simulink model "DTC_Switching"  (R2014a)
settings: Solver=VariableStepDiscrete  StartTime=0.0  StopTime=1  RelTol=1e-3
libraries: powerlib x9, powerlib_meascontrol x1
settings Model: Creator=ninad gaikawad  LastModifiedBy=ninad gaikawad
settings SolverCC: ZeroCrossAlgorithm=Adaptive

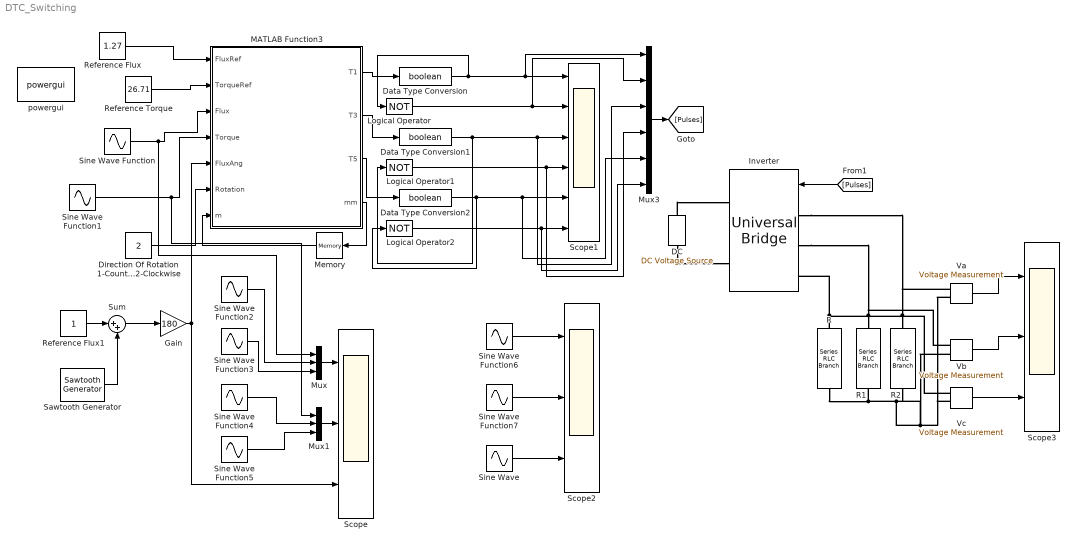
== system DTC_Switching ==
  "DC " : powerlib/Electrical Sources/DC Voltage Source  Amplitude=200  Measurements=None
  Data Type Conversion : DataTypeConversion  OutDataTypeStr=boolean
  Data Type Conversion1 : DataTypeConversion  OutDataTypeStr=boolean
  Data Type Conversion2 : DataTypeConversion  OutDataTypeStr=boolean
  Direction Of Rotation 1-CounterClockwise 2-Clockwise : Constant  Value=2
  Gain : Gain  Gain=180
  Inverter : powerlib/Power Electronics/Universal Bridge  Arms=3  SnubberResistance=1e5  SnubberCapacitance=inf  Device=IGBT / Diodes  Ron=1e-3  Lon=0  ForwardVoltages="[  0  0  ]"  ForwardVoltage=0  GTOparameters=[ 10e-6 , 20e-6 ]  IGBTparameters=[ 1e-6 , 2e-6 ]  Measurements=None  Measurements_2=None  converterType=Rectifier
  Logical Operator : Logic  Operator=NOT  AllPortsSameDT=off  OutDataTypeStr=boolean
  Logical Operator1 : Logic  Operator=NOT  AllPortsSameDT=off  OutDataTypeStr=boolean
  Logical Operator2 : Logic  Operator=NOT  AllPortsSameDT=off  OutDataTypeStr=boolean
  MATLAB Function3 : MATLAB Function  TreatAsAtomicUnit=on
  Memory : Memory  X0=1
  Mux : Mux  Inputs=3
  Mux1 : Mux  Inputs=3
  Mux3 : Mux  Inputs=6
  R : powerlib/Elements/Series RLC Branch  LConnTagsString=__new0  RConnTagsString=__new0  BranchType=R  Resistance=1000  Inductance=1e-3  SetiL0=off  InitialCurrent=0  Capacitance=1e-6  Setx0=off  InitialVoltage=0  Measurements=None
  R1 : powerlib/Elements/Series RLC Branch  LConnTagsString=__new0  RConnTagsString=__new0  BranchType=R  Resistance=1000  Inductance=1e-3  SetiL0=off  InitialCurrent=0  Capacitance=1e-6  Setx0=off  InitialVoltage=0  Measurements=None
  R2 : powerlib/Elements/Series RLC Branch  LConnTagsString=__new0  RConnTagsString=__new0  BranchType=R  Resistance=1000  Inductance=1e-3  SetiL0=off  InitialCurrent=0  Capacitance=1e-6  Setx0=off  InitialVoltage=0  Measurements=None
  Reference Flux : Constant  Value=1.27
  Reference Flux1 : Constant
  Reference Torque : Constant  Value=26.71
  Sawtooth Generator : powerlib_meascontrol/Pulse & Signal Generators/Sawtooth Generator  Freq=50  Phase=0  Ts=0
  Scope : Scope  NumInputPorts=3
      settings: YMin=-5~-5~-5  YMax=5~5~5
  Scope1 : Scope  NumInputPorts=6
      settings: YMin=-5~-5~-5~-5~-5~-5  YMax=5~5~5~5~5~5
  Scope2 : Scope  NumInputPorts=3
      settings: YMin=-5~-5~-5  YMax=5~5~5  SaveName=ScopeData2
  Scope3 : Scope  NumInputPorts=3
      settings: YMin=-5~-5~-5  YMax=5~5~5  SaveName=ScopeData3
  Sine Wave : Sin  Frequency=2*pi*50  SampleTime=0
  Sine Wave Function : Sin  Amplitude=1.3  Bias=1.27  Frequency=2*pi*50  SampleTime=0
  Sine Wave Function1 : Sin  Amplitude=28  Bias=26.71  Frequency=2*pi*50  SampleTime=0
  Sine Wave Function2 : Sin  Amplitude=1.3+0.025  Bias=1.27+0.025  Frequency=2*pi*50  SampleTime=0
  Sine Wave Function3 : Sin  Amplitude=1.3-0.025  Bias=1.27-0.025  Frequency=2*pi*50  SampleTime=0
  Sine Wave Function4 : Sin  Amplitude=26.71+0.25  Bias=26.71+0.25  Frequency=2*pi*50  SampleTime=0
  Sine Wave Function5 : Sin  Amplitude=26.71-0.25  Bias=26.71-0.25  Frequency=2*pi*50  SampleTime=0
  Sine Wave Function6 : Sin  Amplitude=1.3  Bias=1.27  Frequency=2*pi*50  SampleTime=0
  Sine Wave Function7 : Sin  Amplitude=28  Bias=26.71  Frequency=2*pi*50  SampleTime=0
  Sum : Sum  Inputs=|++
  Va : powerlib/Measurements/Voltage Measurement  PhasorSimulation=off  OutputType=Complex  PSBequivalent=0
  Vb : powerlib/Measurements/Voltage Measurement  PhasorSimulation=off  OutputType=Complex  PSBequivalent=0
  Vc : powerlib/Measurements/Voltage Measurement  PhasorSimulation=off  OutputType=Complex  PSBequivalent=0
  powergui : powerlib/powergui  Priority=1  SimulationMode=Discrete  SolverType=Tustin  SampleTime=50e-6  frequency=60  SPID=off  DisableSnubberDevices=off  DisableRonSwitches=off  DisableVfSwitches=off  SwTol=0  Interpol=off  DisplayEquations=off  Ts=0  methode=off  frequencyindice=0  Pbase=100e6  ErrMax=1e-4  Iterations=50  UnitsV=kV  UnitsW=MW  FunctionMessages=off  echomessages=off  HookPort=off  EnableUseOfTLC=off  x0status=blocks  RestoreLinks=warning  ResistiveCurrentMeasurement=off  Frange=[0:2:500]  Ylog=off  Xlog=on  ShowGrid=off  save=off  variable=ZData  structure=0  ZoomFFT=off  StartTime=0.0  cycles=1  DisplayStyle=1  fundamental=60  FreqAxis=off  MaxFrequency=1000  frequencyindicesteady=1  RmsSteady=1  display=off
  wires:
  Sine Wave Function/1 -> Mux/1, MATLAB Function3/3(Flux)
  Sine Wave Function1/1 -> MATLAB Function3/4(Torque), Mux1/1
  Reference Flux/1 -> MATLAB Function3/1(FluxRef)
  Reference Torque/1 -> MATLAB Function3/2(TorqueRef)
  Direction Of Rotation 1-CounterClockwise 2-Clockwise/1 -> MATLAB Function3/6(Rotation)
  MATLAB Function3/1(T1) -> Data Type Conversion/1
  MATLAB Function3/2(T3) -> Data Type Conversion1/1
  MATLAB Function3/3(T5) -> Data Type Conversion2/1
  Logical Operator/1 -> Mux3/2, Scope1/2
  Logical Operator2/1 -> Mux3/6, Scope1/6
  Data Type Conversion/1 -> Logical Operator/1, Mux3/1, Scope1/1
  Data Type Conversion2/1 -> Logical Operator2/1, Mux3/5, Scope1/5
  Data Type Conversion1/1 -> Logical Operator1/1, Mux3/3, Scope1/3
  MATLAB Function3/4(mm) -> Memory/1
  Memory/1 -> MATLAB Function3/7(m)
  Reference Flux1/1 -> Sum/1
  Sawtooth Generator/1 -> Sum/2
  Sum/1 -> Gain/1
  Gain/1 -> MATLAB Function3/5(FluxAng), Scope/3
  Mux/1 -> Scope/1
  Mux1/1 -> Scope/2
  Sine Wave Function2/1 -> Mux/2
  Sine Wave Function3/1 -> Mux/3
  Sine Wave Function4/1 -> Mux1/2
  Sine Wave Function5/1 -> Mux1/3
  Sine Wave Function7/1 -> Scope2/2
  Sine Wave Function6/1 -> Scope2/1
  Sine Wave/1 -> Scope2/3
  Va/1 -> Scope3/1
  Vb/1 -> Scope3/2
  Vc/1 -> Scope3/3
  Logical Operator1/1 -> Mux3/4, Scope1/4
  [Pulses] -> Inverter/1
  Mux3/1 -> [Pulses]
  connections:
  Vc/LConn1 -- R/LConn1 -- Inverter/LConn3
  R1/LConn1 -- Inverter/LConn2 -- Vb/LConn1
  R2/LConn1 -- Inverter/LConn1 -- Va/LConn1
  R1/RConn1 -- R/RConn1 -- R2/RConn1 -- Vb/LConn2 -- Va/LConn2 -- Vc/LConn2
  "DC "/RConn1 -- Inverter/RConn1
  "DC "/LConn1 -- Inverter/RConn2

== matlab function DTC_Switching/MATLAB Function3 ==
  settings: updateMethod=CONTINUOUS
  data: FluxRef input; TorqueRef input; Flux input; Torque input; T1 output; T3 output; FluxAng input; T5 output; Rotation input; m input; mm output
function [T1,T3,T5,mm] = DTC_SwitchingTable(FluxRef,TorqueRef,Flux,Torque,FluxAng,Rotation,m)
 
T1=0;
T3=0;
T5=0;

DelF=0.025;% Hysteresis Width for Flux
DelT=0.25;% Hysteresis Width for Torque

Hf=0;%Initializing Hysteresis Controller Output For Flux
Ht=0;%Initializing Hysteresis Controller Output For Torque
S=0;%Initializing DTC Space Vector Sector
mm=m;
% Flux Two Level Hysteresis Band %
%------------------------------------------------------------------------%
if(Flux<=(FluxRef-DelF))
    Hf=1;
    mm=Hf;
end
if(mm==1&&(Flux>(FluxRef-DelF)&&Flux<(FluxRef+DelF)))
    Hf=1;
    mm=Hf;
end
if(Flux>=(FluxRef+DelF))
    Hf=0;
    mm=Hf;
end
if(mm==0&&(Flux>(FluxRef-DelF)&&Flux<(FluxRef+DelF)))
    Hf=0;
    mm=Hf;
end

% Torque Three Level Hysteresis Band %
%------------------------------------------------------------------------%
if(Torque<=(TorqueRef-DelT))
    Ht=1;
end
if(Torque>(TorqueRef-DelT)&&Torque<(TorqueRef+DelT))
    Ht=0;
end
if(Torque>=(TorqueRef+DelT))
    Ht=-1;
end

% DTC Sector Prediction %
%------------------------------------------------------------------------%
if(FluxAng>=330&&FluxAng<30)
    S=1;
end
if(FluxAng>=30&&FluxAng<90)
    S=2;
end
if(FluxAng>=90&&FluxAng<150)
    S=3;
end
if(FluxAng>=150&&FluxAng<210)
    S=4;
end
if(FluxAng>=210&&FluxAng<270)
    S=5;
end
if(FluxAng>=270&&FluxAng<330)
    S=6;
end

% Voltage Vector Synthesis %
%------------------------------------------------------------------------%
if(Rotation==2)% Clockwise Rotation
%------------------------------------------------------------------------%    
    if(Hf==1&&Ht==1&&S==1)
        T1=1;
        T3=0;
        T5=1;
    end
    if(Hf==1&&Ht==1&&S==2)
      T1=0;
      T3=0;
      T5=1;  
    end
    if(Hf==1&&Ht==1&&S==3)
      T1=0;
      T3=1;
      T5=1; 
    end
    if(Hf==1&&Ht==1&&S==4)
      T1=0;
      T3=1;
      T5=0;
    end
    if(Hf==1&&Ht==1&&S==5)
      T1=1;
      T3=1;
      T5=0;    
    end
    if(Hf==1&&Ht==1&&S==6)
      T1=1;
      T3=0;
      T5=0;
    end
   
%------------------------------------------------------------------------%    
    if(Hf==1&&Ht==0&&S==1)
        T1=1;
        T3=1;
        T5=1;
    end
    if(Hf==1&&Ht==0&&S==2)
      T1=0;
      T3=0;
      T5=0;  
    end
    if(Hf==1&&Ht==0&&S==3)
      T1=1;
      T3=1;
      T5=1; 
    end
    if(Hf==1&&Ht==0&&S==4)
      T1=0;
      T3=0;
      T5=0;
    end
    if(Hf==1&&Ht==0&&S==5)
      T1=1;
      T3=1;
      T5=1;    
    end
    if(Hf==1&&Ht==0&&S==6)
      T1=0;
      T3=0;
      T5=0;
    end
%------------------------------------------------------------------------%    
    if(Hf==1&&Ht==-1&&S==1)
        T1=1;
        T3=1;
        T5=0;
    end
    if(Hf==1&&Ht==-1&&S==2)
      T1=1;
      T3=0;
      T5=0;  
    end
    if(Hf==1&&Ht==-1&&S==3)
      T1=1;
      T3=0;
      T5=1; 
    end
    if(Hf==1&&Ht==-1&&S==4)
      T1=0;
      T3=0;
      T5=1;
    end
    if(Hf==1&&Ht==-1&&S==5)
      T1=0;
      T3=1;
      T5=1;    
    end
    if(Hf==1&&Ht==-1&&S==6)
      T1=0;
      T3=1;
      T5=0;
    end
    
 %------------------------------------------------------------------------%   
    
     if(Hf==0&&Ht==1&&S==1)
        T1=0;
        T3=0;
        T5=1;
    end
    if(Hf==0&&Ht==1&&S==2)
      T1=0;
      T3=1;
      T5=1;  
    end
    if(Hf==0&&Ht==1&&S==3)
      T1=0;
      T3=1;
      T5=0; 
    end
    if(Hf==0&&Ht==1&&S==4)
      T1=1;
      T3=1;
      T5=0;
    end
    if(Hf==0&&Ht==1&&S==5)
      T1=1;
      T3=0;
      T5=0;    
    end
    if(Hf==0&&Ht==1&&S==6)
      T1=1;
      T3=0;
      T5=1;
    end
%------------------------------------------------------------------------%    
    
    if(Hf==0&&Ht==0&&S==1)
        T1=0;
        T3=0;
        T5=0;
    end
    if(Hf==0&&Ht==0&&S==2)
      T1=1;
      T3=1;
      T5=1;  
    end
    if(Hf==0&&Ht==0&&S==3)
      T1=0;
      T3=0;
      T5=0; 
    end
    if(Hf==0&&Ht==0&&S==4)
      T1=1;
      T3=1;
      T5=1;
    end
    if(Hf==0&&Ht==0&&S==5)
      T1=0;
      T3=0;
      T5=0;    
    end
    if(Hf==0&&Ht==0&&S==6)
      T1=1;
      T3=1;
      T5=1;
    end
  %------------------------------------------------------------------------%  
    
    if(Hf==0&&Ht==-1&&S==1)
        T1=0;
        T3=1;
        T5=0;
    end
    if(Hf==0&&Ht==-1&&S==2)
      T1=1;
      T3=1;
      T5=0;  
    end
    if(Hf==0&&Ht==-1&&S==3)
      T1=1;
      T3=0;
      T5=0; 
    end
    if(Hf==0&&Ht==-1&&S==4)
      T1=1;
      T3=0;
      T5=1;
    end
    if(Hf==0&&Ht==-1&&S==5)
      T1=0;
      T3=0;
      T5=1;    
    end
    if(Hf==0&&Ht==-1&&S==6)
      T1=0;
      T3=1;
      T5=1;
    end
end

%------------------------------------------------------------------------%
if(Rotation==1)% Counter-Clockwise Rotation
%------------------------------------------------------------------------%    
    if(Hf==1&&Ht==1&&S==1)
        T1=1;
        T3=1;
        T5=0;
    end
    if(Hf==1&&Ht==1&&S==2)
      T1=0;
      T3=1;
      T5=0;  
    end
    if(Hf==1&&Ht==1&&S==3)
      T1=0;
      T3=1;
      T5=1; 
    end
    if(Hf==1&&Ht==1&&S==4)
      T1=0;
      T3=0;
      T5=1;
    end
    if(Hf==1&&Ht==1&&S==5)
      T1=1;
      T3=0;
      T5=1;    
    end
    if(Hf==1&&Ht==1&&S==6)
      T1=1;
      T3=0;
      T5=0;
    end
   
%------------------------------------------------------------------------%    
    if(Hf==1&&Ht==0&&S==1)
        T1=1;
        T3=1;
        T5=1;
    end
    if(Hf==1&&Ht==0&&S==2)
      T1=0;
      T3=0;
      T5=0;  
    end
    if(Hf==1&&Ht==0&&S==3)
      T1=1;
      T3=1;
      T5=1; 
    end
    if(Hf==1&&Ht==0&&S==4)
      T1=0;
      T3=0;
      T5=0;
    end
    if(Hf==1&&Ht==0&&S==5)
      T1=1;
      T3=1;
      T5=1;    
    end
    if(Hf==1&&Ht==0&&S==6)
      T1=0;
      T3=0;
      T5=0;
    end
%------------------------------------------------------------------------%    
    if(Hf==1&&Ht==-1&&S==1)
        T1=1;
        T3=0;
        T5=1;
    end
    if(Hf==1&&Ht==-1&&S==2)
      T1=1;
      T3=0;
      T5=0;  
    end
    if(Hf==1&&Ht==-1&&S==3)
      T1=1;
      T3=1;
      T5=0; 
    end
    if(Hf==1&&Ht==-1&&S==4)
      T1=0;
      T3=1;
      T5=0;
    end
    if(Hf==1&&Ht==-1&&S==5)
      T1=0;
      T3=1;
      T5=1;    
    end
    if(Hf==1&&Ht==-1&&S==6)
      T1=0;
      T3=0;
      T5=1;
    end
    
 %------------------------------------------------------------------------%   
    
     if(Hf==0&&Ht==1&&S==1)
        T1=0;
        T3=1;
        T5=0;
    end
    if(Hf==0&&Ht==1&&S==2)
      T1=0;
      T3=1;
      T5=1;  
    end
    if(Hf==0&&Ht==1&&S==3)
      T1=0;
      T3=0;
      T5=1; 
    end
    if(Hf==0&&Ht==1&&S==4)
      T1=1;
      T3=0;
      T5=1;
    end
    if(Hf==0&&Ht==1&&S==5)
      T1=1;
      T3=0;
      T5=0;    
    end
    if(Hf==0&&Ht==1&&S==6)
      T1=1;
      T3=1;
      T5=0;
    end
%------------------------------------------------------------------------%    
    
    if(Hf==0&&Ht==0&&S==1)
        T1=0;
        T3=0;
        T5=0;
    end
    if(Hf==0&&Ht==0&&S==2)
      T1=1;
      T3=1;
      T5=1;  
    end
    if(Hf==0&&Ht==0&&S==3)
      T1=0;
      T3=0;
      T5=0; 
    end
    if(Hf==0&&Ht==0&&S==4)
      T1=1;
      T3=1;
      T5=1;
    end
    if(Hf==0&&Ht==0&&S==5)
      T1=0;
      T3=0;
      T5=0;    
    end
    if(Hf==0&&Ht==0&&S==6)
      T1=1;
      T3=1;
      T5=1;
    end
  %------------------------------------------------------------------------%  
    
    if(Hf==0&&Ht==-1&&S==1)
        T1=0;
        T3=0;
        T5=1;
    end
    if(Hf==0&&Ht==-1&&S==2)
      T1=1;
      T3=0;
      T5=1;  
    end
    if(Hf==0&&Ht==-1&&S==3)
      T1=1;
      T3=0;
      T5=0; 
    end
    if(Hf==0&&Ht==-1&&S==4)
      T1=1;
      T3=1;
      T5=0;
    end
    if(Hf==0&&Ht==-1&&S==5)
      T1=0;
      T3=1;
      T5=0;    
    end
    if(Hf==0&&Ht==-1&&S==6)
      T1=0;
      T3=1;
      T5=1;
    end
end
